simulink model "untitled2"  (R2018b)
settings: Solver=VariableStepAuto  StartTime=0.0  StopTime=10.0  RelTol=1e-3
libraries: dsparch4 x2
settings Model: Creator=nhat  LastModifiedBy=nhat

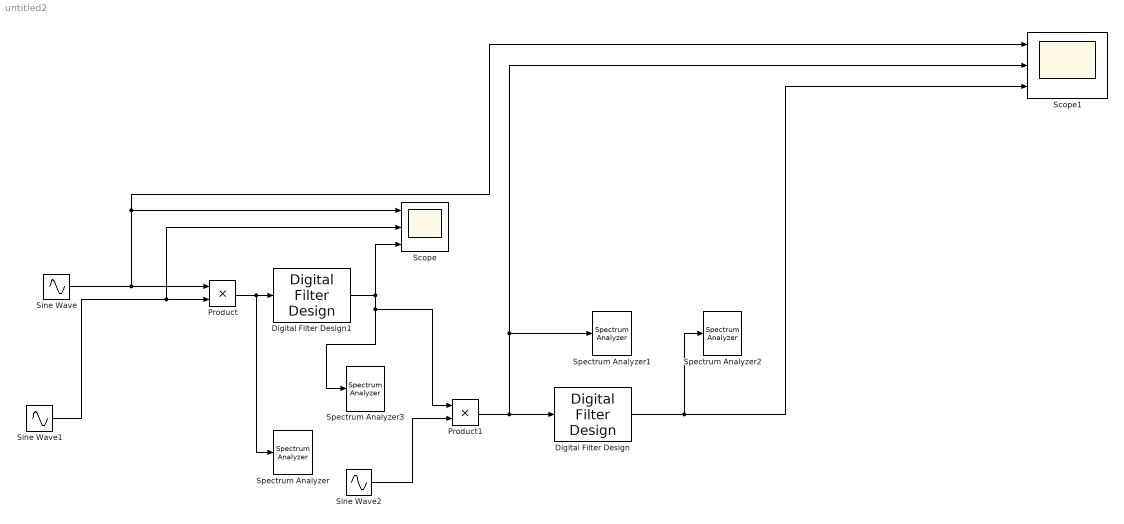
== system untitled2 ==
  Digital Filter Design : dsparch4/Digital Filter Design  mwdsp_browser_bugfix_var=off
  Digital Filter Design1 : dsparch4/Digital Filter Design  mwdsp_browser_bugfix_var=off
  Product : Product
  Product1 : Product
  Scope : Scope  NumInputPorts=3
  Scope1 : Scope  NumInputPorts=3
  Sine Wave : Sin  Frequency=1000*2*pi  SampleTime=1/100000
  Sine Wave1 : Sin  Amplitude=5  Frequency=10000*2*pi  SampleTime=1/100000
  Sine Wave2 : Sin  Amplitude=5  Frequency=10000*2*pi  SampleTime=1/100000
  Spectrum Analyzer{,1..3} (4 alike) : SpectrumAnalyzer
  wires:
  Sine Wave1/1 -> Scope/2, Product/2
  Sine Wave2/1 -> Product1/2
  Sine Wave/1 -> Product/1, Scope1/1, Scope/1
  Product1/1 -> Scope1/2, Spectrum Analyzer1/1, Digital Filter Design/1
  Digital Filter Design/1 -> Scope1/3, Spectrum Analyzer2/1
  Product/1 -> Spectrum Analyzer/1, Digital Filter Design1/1
  Digital Filter Design1/1 -> Product1/1, Spectrum Analyzer3/1, Scope/3
